simulink model "openLoopTest"  (R2021a)
settings: Solver=FixedStepAuto  StartTime=0.0  StopTime=3  FixedStep=0.001  RelTol=1e-3  EnableMultiTasking=on
libraries: arduinolib x2
settings Model: SILPILModeSetting=veronly  ExtModeTrigDuration=2  Creator=s269684  LastModifiedBy=s269684
settings OptimizationCC: EnhancedBackFolding=on  PassReuseOutputArgsAs=Individual arguments  ZeroExternalMemoryAtStartup=off  ZeroInternalMemoryAtStartup=off  MaxStackSize=64  OptimizeBlockOrder=speed  DifferentSizesBufferReuse=on  OptimizationCustomize=off  EfficientTunableParamExpr=on
settings DebuggingCC: ParameterTunabilityLossMsg=error
settings HardwareCC: ProdBitPerInt=16  ProdBitPerPointer=16  ProdBitPerSizeT=16  ProdBitPerPtrDiffT=16  ProdLargestAtomicFloat=None  ProdWordSize=8  ProdHWDeviceType=Atmel->AVR  UseEmbeddedCoderFeatures=off
settings SFSimCC: MATLABDynamicMemAlloc=off
settings RTWCC: SystemTargetFile=ert.tlc  HardwareBoard=Arduino Uno  TemplateMakefile=ert_default_tmf  Toolchain=Arduino AVR  BuildConfiguration=Faster Runs
settings CodeAppCC: ForceParamTrailComments=on  IgnoreCustomStorageClasses=off  OperatorAnnotations=on  SimulinkDataObjDesc=on  SFDataObjDesc=on  InsertBlockDesc=on
settings ERTTargetCC: SupportContinuousTime=on  SupportNonInlinedSFcns=on  SupportVariableSizeSignals=on  ExtModeTransport=3  ExtModeStaticAlloc=on  ExtModeStaticAllocSize=250  ExtModeMexFile=ext_xcp  ExtModeIntrfLevel=Level2 - Open

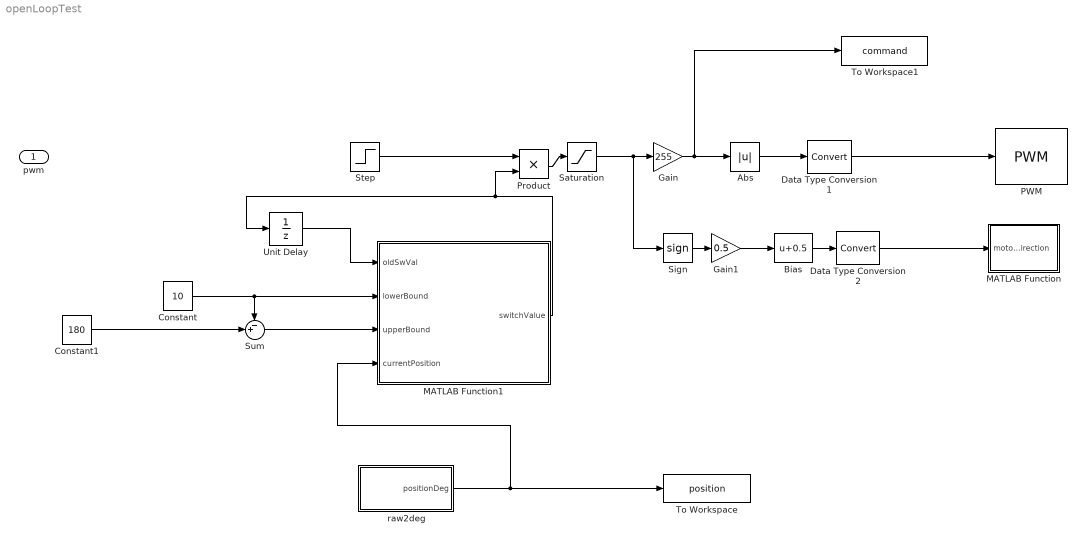
== system openLoopTest ==
  pwm : Inport
  Abs : Abs
  Bias : Bias  Bias=0.5
  Constant : Constant  Value=10
  Constant1 : Constant  Value=180
  Data Type Conversion1 : DataTypeConversion
  Data Type Conversion2 : DataTypeConversion
  Gain : Gain  Gain=255
  Gain1 : Gain  Gain=0.5
  MATLAB Function : MATLAB Function  TreatAsAtomicUnit=on
  MATLAB Function1 : MATLAB Function  TreatAsAtomicUnit=on
  PWM : arduinolib/PWM  pinNumber=6  frequencyType=Default  desiredFrequency=490.2  achievableFrequency=490.2
  Product : Product
  Saturation : Saturate  UpperLimit=1  LowerLimit=-1
  Sign : Signum
  Step : Step  After=-1  SampleTime=0
  Sum : Sum  Inputs=-+|
  To Workspace : ToWorkspace  VariableName=position  SaveFormat=Structure With Time  SampleTime=-1
  To Workspace1 : ToWorkspace  VariableName=command  SaveFormat=Structure With Time  SampleTime=-1
  Unit Delay : UnitDelay  InitialCondition=1  SampleTime=-1  HasFrameUpgradeWarning=on
  raw2deg : Subsystem
  wires:
  raw2deg/1(positionDeg) -> MATLAB Function1/4(currentPosition), To Workspace/1
  Data Type Conversion2/1 -> MATLAB Function/1(motorDirection)
  Sign/1 -> Gain1/1
  Saturation/1 -> Sign/1, Gain/1
  Step/1 -> Product/1
  Abs/1 -> Data Type Conversion1/1
  Data Type Conversion1/1 -> PWM/1
  Gain1/1 -> Bias/1
  Bias/1 -> Data Type Conversion2/1
  Gain/1 -> To Workspace1/1, Abs/1
  Unit Delay/1 -> MATLAB Function1/1(oldSwVal)
  MATLAB Function1/1(switchValue) -> Product/2, Unit Delay/1
  Constant/1 -> Sum/1, MATLAB Function1/2(lowerBound)
  Constant1/1 -> Sum/2
  Product/1 -> Saturation/1
  Sum/1 -> MATLAB Function1/3(upperBound)

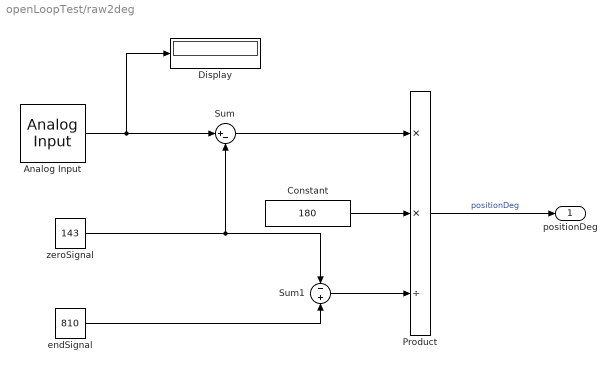
== system openLoopTest/raw2deg ==
  Analog Input : arduinolib/Analog Input  pinNumber=1  ReadResultsOnly=off  ConversionTriggerSource=Software  ExternalTriggerType=uint32( 0 )  OutputDataType=uint16  EnableConversionCompleteNotify=off  EnableOuputStatus=off  SampleTime=-1  blockPlatform=arduino
  Constant : Constant  Value=180
  Display : Display
  Product : Product  Inputs=**/
  Sum : Sum  Inputs=|+-
  Sum1 : Sum  Inputs=-+
  endSignal : Constant  Value=810
  zeroSignal : Constant  Value=143
  positionDeg : Outport
  wires:
  Sum1/1 -> Product/3
  Analog Input/1 -> Display/1, Sum/1
  zeroSignal/1 -> Sum1/1, Sum/2
  endSignal/1 -> Sum1/2
  Sum/1 -> Product/1
  Constant/1 -> Product/2
  Product/1 -> positionDeg/1  "positionDeg"

== matlab function openLoopTest/MATLAB Function1 ==
  data: oldSwVal input; switchValue output; lowerBound input; upperBound input; currentPosition input
function switchValue = inputGuard(oldSwVal, lowerBound, upperBound, currentPosition)
if currentPosition > lowerBound && currentPosition<upperBound
    switchValue = oldSwVal;
else
    switchValue = 0;
end

== matlab function openLoopTest/MATLAB Function ==
  data: motorDirection input
function fcn(motorDirection)
persistent arduinoObj;
directionPin = "A0";
if (isempty(arduinoObj))
    arduinoObj = arduino();
    arduinoObj.configurePin(directionPin , "DigitalOutput");
end

arduinoObj.writeDigitalPin(directionPin, motorDirection)
end
